simulink model "schemat_nieliniowy"  (R2015a)
settings: Solver=ode45  StartTime=0.0  StopTime=4000  MaxStep=400  RelTol=1e-3
values from neighbouring files (symbols this model uses):
  cp = 1000    [mini_projekt_6b_baza.m]    (also in symulacje_bez_simulinka.m)
  Cvp = cp * rop * Vp    (= 1500000)    [mini_projekt_6b_baza.m]    (also in symulacje_bez_simulinka.m)
  Cvw = cp * rop * Vw    (= 3000000)    [mini_projekt_6b_baza.m]    (also in symulacje_bez_simulinka.m)
  dfk = 0*fk    (= 0)    [mini_projekt_6b_baza.m]
  dTkz = 0    [mini_projekt_6b_baza.m]    (also in symulacje_bez_simulinka.m = 2)
  dTzew = 0    [mini_projekt_6b_baza.m]    (also in symulacje_bez_simulinka.m = 2)
  fko = fk    (= 0.47619047619)    [mini_projekt_6b_baza.m]
  K1 = (0.6*cp*rop*fk*(Tkzn-Twewn))/(Twewn - Tzewn)    (= 128.571428571)    [mini_projekt_6b_baza.m]    (also in symulacje_bez_simulinka.m)
  K2 = X(1)    [mini_projekt_6b_baza.m]    (also in symulacje_bez_simulinka.m)
  Kp = X(2)    [mini_projekt_6b_baza.m]    (also in symulacje_bez_simulinka.m)
  rop = 1.2    [mini_projekt_6b_baza.m]    (also in symulacje_bez_simulinka.m)
  t0 = 5000    [mini_projekt_6b_baza.m]    (also in symulacje_bez_simulinka.m)
  Tkzo = Tkzn    (= 35)    [mini_projekt_6b_baza.m]
  Tpo1 = M*(Kp*Twewo1+K2*Tzewo)    [mini_projekt_6b_baza.m]
  Twewo1 = (cpf*Tkzo+K1*Tzewo+Kp*K2*M*Tzewo)/(cpf+K1+Kp-M*Kp^2)    [mini_projekt_6b_baza.m]
  Tzewo = Tzewn    (= -20)    [mini_projekt_6b_baza.m]
settings Model: Creator=LAB320-1552  LastModifiedBy=apuch
settings DataIOCC: SignalLoggingSaveFormat=ModelDataLogs
settings DebuggingCC: UnderspecifiedInitializationDetection=Classic  MergeDetectMultiDrivingBlocksExec=none  SolverPrmCheckMsg=warning  MultiTaskDSMMsg=warning  MultiTaskCondExecSysMsg=none  StateNameClashWarn=warning

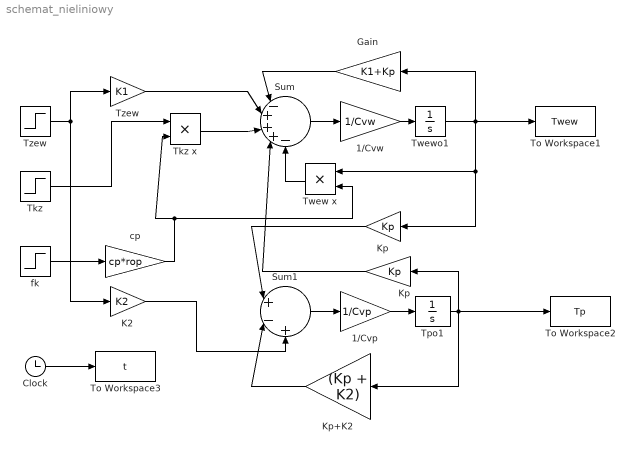
== system schemat_nieliniowy ==
  1/Cvp : Gain  Gain=1/Cvp
  1/Cvw : Gain  Gain=1/Cvw
  Clock : Clock
  Gain : Gain  Gain=K1+Kp
  K2 : Gain  Gain=K2
  Kp : Gain  Gain=Kp
  "Kp " : Gain  Gain=Kp
  Kp+K2 : Gain  Gain=(Kp + K2)
  Sum : Sum  Inputs=|-+++-
  Sum1 : Sum  Inputs=|+-+
  Tkz : Step  Time=t0  Before=Tkzo  After=Tkzo + dTkz  SampleTime=0
  Tkz x : Product
  To Workspace1 : ToWorkspace  VariableName=Twew  SampleTime=-1
  To Workspace2 : ToWorkspace  VariableName=Tp  SampleTime=-1
  To Workspace3 : ToWorkspace  VariableName=t  SampleTime=-1
  Tpo1 : Integrator  InitialCondition=Tpo1
  Twew x : Product
  Twewo1 : Integrator  InitialCondition=Twewo1
  Tzew : Step  Time=t0  Before=Tzewo  After=Tzewo + dTzew  SampleTime=0
  "Tzew " : Gain  Gain=K1
  "cp " : Gain  Gain=cp*rop
  fk : Step  Time=t0  Before=fko  After=fko + dfk  SampleTime=0
  wires:
  Tzew/1 -> K2/1, "Tzew "/1
  "Tzew "/1 -> Sum/2
  Sum/1 -> 1/Cvw/1
  1/Cvw/1 -> Twewo1/1
  Twewo1/1 -> Twew x/1, Kp/1, Gain/1, To Workspace1/1
  "Kp "/1 -> Sum/4
  Tpo1/1 -> "Kp "/1, Kp+K2/1, To Workspace2/1
  Clock/1 -> To Workspace3/1
  1/Cvp/1 -> Tpo1/1
  Sum1/1 -> 1/Cvp/1
  K2/1 -> Sum1/3
  Kp+K2/1 -> Sum1/2
  Kp/1 -> Sum1/1
  fk/1 -> "cp "/1
  Tkz/1 -> Tkz x/1
  Tkz x/1 -> Sum/3
  Twew x/1 -> Sum/5
  "cp "/1 -> Tkz x/2, Twew x/2
  Gain/1 -> Sum/1
